simulink model "PrinterILC_exp"  (Simulink 7.8)
settings: Solver=FixedStepDiscrete  StartTime=0.0  StopTime=30  FixedStep=1/1000  RelTol=1e-3
undefined symbols (not defined in the file or in its folder): DiscIntNeverNeededParam
libraries: simulink x3
settings Model: Creator=root  LastModifiedBy=root  SimulationMode=external  ExtModeAutoUpdateStatusClock=off
settings DataIOCC: SaveOutput=off  SignalLogging=off  DSMLogging=off  SaveTime=off
settings OptimizationCC: InitFltsAndDblsToZero=on
settings DebuggingCC: SaveWithParameterizedLinksMsg=none  SignalResolutionControl=TryResolveAllWithWarning  MultiTaskDSMMsg=warning  MultiTaskCondExecSysMsg=none  FcnCallInpInsideContextMsg=Use local settings  StrictBusMsg=None
settings SFSimCC: SFSimEcho=off  SimBuildMode=sf_nonincremental_build
settings RTWCC: SystemTargetFile=ectarget.tlc  MakeCommand="make_rtw OPTS=\"-DNETIF_ID=0\""  TemplateMakefile=ec_unix.tmf  Description=Ethercattarget Real-Time Target for PREEMPT-RT/Linux  ProcessScript=ectarget_make_rtw_hook  IncludeERTFirstTime=on  RTWCompilerOptimization=On
settings CodeAppCC: GenerateComments=off  SimulinkBlockComments=off
settings GRTTargetCC: TargetFcnLib=ansi_tfl_tmw.mat  ExtMode=on

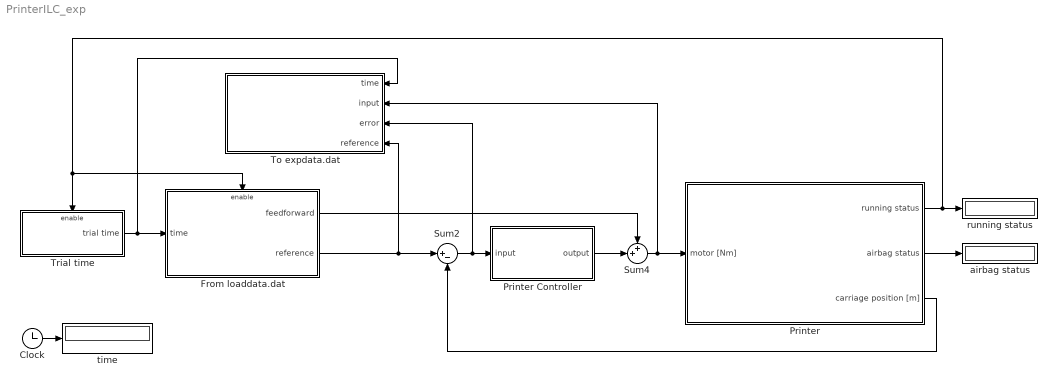
== system PrinterILC_exp ==
  Clock : Clock
  From loaddata.dat : Subsystem
  Printer : Subsystem
  Printer Controller : Subsystem
  Sum2 : Sum  Inputs=|+-
  Sum4 : Sum  Inputs=++|  SaturateOnIntegerOverflow=on  InputSameDT=on  OutDataTypeStr=Inherit: Same as first input
  To expdata.dat : Subsystem
  Trial time : Subsystem  TreatAsAtomicUnit=on
  airbag status : Display
      settings: Decimation=50
  running status : Display
      settings: Decimation=50
  time : Display
      settings: Decimation=50
  wires:
  Sum2/1 -> To expdata.dat/3(error), Printer Controller/1(input)
  From loaddata.dat/2(reference) -> Sum2/1, To expdata.dat/4(reference)
  Clock/1 -> time/1
  Printer/3(carriage position [m]) -> Sum2/2
  Printer Controller/1(output) -> Sum4/2
  From loaddata.dat/1(feedforward) -> Sum4/1
  Sum4/1 -> Printer/1(motor [Nm]), To expdata.dat/2(input)
  Printer/1(running status) -> Trial time/Enable, From loaddata.dat/Enable, running status/1
  Trial time/1(trial time) -> From loaddata.dat/1(time), To expdata.dat/1(time)
  Printer/2(airbag status) -> airbag status/1

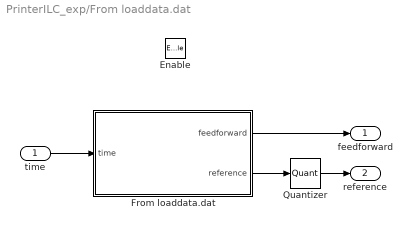
== system PrinterILC_exp/From loaddata.dat ==
  time : Inport
  Enable : EnablePort  StatesWhenEnabling=reset
  From loaddata.dat : Subsystem
  Quantizer : Quantizer  QuantizationInterval=1/(600*100/2.54)
  feedforward : Outport
  reference : Outport  Port=2
  wires:
  time/1 -> From loaddata.dat/1(time)
  From loaddata.dat/1(feedforward) -> feedforward/1
  From loaddata.dat/2(reference) -> Quantizer/1
  Quantizer/1 -> reference/1

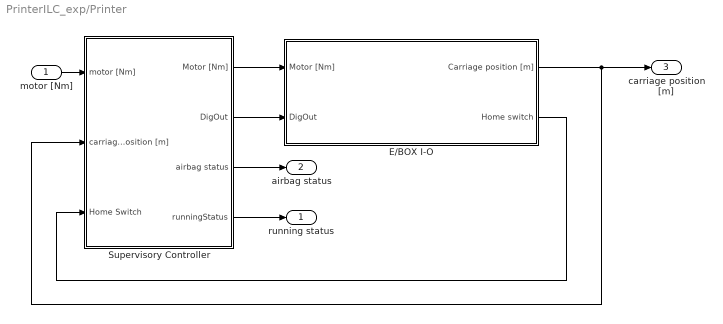
== system PrinterILC_exp/Printer ==
  motor [Nm] : Inport
  E/BOX I-O : Subsystem
  Supervisory Controller : Subsystem
  running status : Outport
  airbag status : Outport  Port=2
  carriage position [m] : Outport  Port=3
  wires:
  E/BOX I-O/1(Carriage position [m]) -> Supervisory Controller/2(carriage position [m]), carriage position [m]/1
  Supervisory Controller/1(Motor [Nm]) -> E/BOX I-O/1(Motor [Nm])
  E/BOX I-O/2(Home switch) -> Supervisory Controller/3(Home Switch)
  motor [Nm]/1 -> Supervisory Controller/1(motor [Nm])
  Supervisory Controller/3(airbag status) -> airbag status/1
  Supervisory Controller/4(runningStatus) -> running status/1
  Supervisory Controller/2(DigOut) -> E/BOX I-O/2(DigOut)

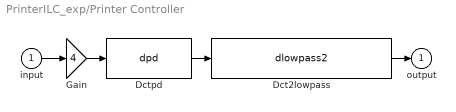
== system PrinterILC_exp/Printer Controller ==
  input : Inport
  Dct2lowpass : S-Function  FunctionName=dlowpass2  Parameters=f_den, b_den, 0.001  EnableBusSupport=off  mask(dctools){f_den=40, b_den=0.7}
      mask prompts: f_den "Pole [Hz]"; b_den "Damping pole [-]"
      mask help: This block implements a discrete time 2nd order lowpass filter.
      mask Display: disp('DCT 2nd order lowpass')
  Dctpd : S-Function  FunctionName=dpd  Parameters=kp, kv, 0.001  EnableBusSupport=off  mask(dctools){kp=40, kv=1}
      mask help: This block implements a discrete time pd filter.
      mask Display: disp('DCT pd')
  Gain : Gain  Gain=4  SaturateOnIntegerOverflow=on  OutDataTypeStr=Inherit: Same as input  ParamDataTypeStr=Inherit: Same as input
  output : Outport
  wires:
  input/1 -> Gain/1
  Gain/1 -> Dctpd/1
  Dctpd/1 -> Dct2lowpass/1
  Dct2lowpass/1 -> output/1

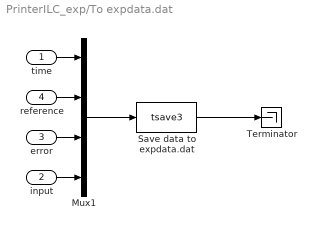
== system PrinterILC_exp/To expdata.dat ==
  time : Inport
  input : Inport  Port=2
  error : Inport  Port=3
  reference : Inport  Port=4
  Mux1 : Mux
  Save data to expdata.dat : S-Function  FunctionName=tsave3  Parameters=0  EnableBusSupport=off
  Terminator : Terminator
  wires:
  Mux1/1 -> Save data to expdata.dat/1
  Save data to expdata.dat/1 -> Terminator/1
  time/1 -> Mux1/1
  input/1 -> Mux1/4
  error/1 -> Mux1/3
  reference/1 -> Mux1/2

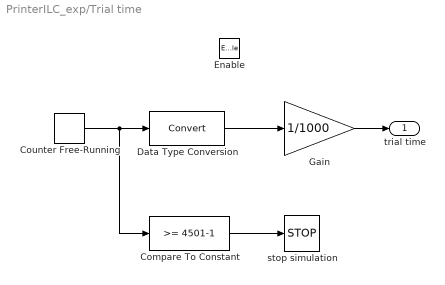
== system PrinterILC_exp/Trial time ==
  Enable : EnablePort  StatesWhenEnabling=reset
  Compare To Constant : simulink/Logic and Bit Operations/Compare To Constant  relop=>=  const=4501-1  OutDataTypeStr=boolean
  Counter Free-Running : simulink/Sources/Counter Free-Running  NumBits=32  tsamp=-1
  Data Type Conversion : DataTypeConversion
  Gain : Gain  Gain=1/1000
  stop simulation : Stop
  trial time : Outport  InitialOutput=0
  wires:
  Counter Free-Running/1 -> Compare To Constant/1, Data Type Conversion/1
  Compare To Constant/1 -> stop simulation/1
  Data Type Conversion/1 -> Gain/1
  Gain/1 -> trial time/1

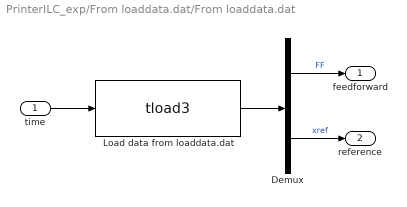
== system PrinterILC_exp/From loaddata.dat/From loaddata.dat ==
  time : Inport
  Demux : Demux  Outputs=2
  Load data from loaddata.dat : S-Function  FunctionName=tload3  Parameters=0  EnableBusSupport=off
  feedforward : Outport
  reference : Outport  Port=2
  wires:
  time/1 -> Load data from loaddata.dat/1
  Load data from loaddata.dat/1 -> Demux/1
  Demux/1 -> feedforward/1  "FF"
  Demux/2 -> reference/1  "xref"

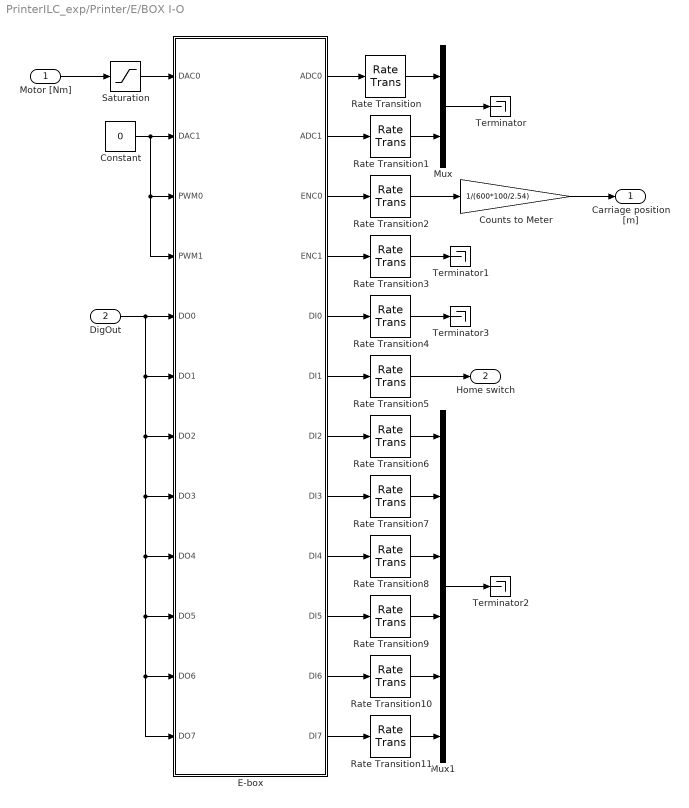
== system PrinterILC_exp/Printer/E/BOX I-O ==
  Motor [Nm] : Inport
  DigOut : Inport  Port=2
  Constant : Constant  Value=0
  Counts to Meter : Gain  Gain=1/(600*100/2.54)
  E-box : Subsystem  mask(E-box){link_id=0}
      mask prompts: link_id "Link id (>=0)"
  Mux : Mux  Inputs=2
  Mux1 : Mux  Inputs=6
  Rate Transition{,1..11} (12 alike) : RateTransition
  Saturation : Saturate  UpperLimit=2.5  LowerLimit=-2.5
  Terminator{,1..3} (4 alike) : Terminator
  Carriage position [m] : Outport
  Home switch : Outport  Port=2
  wires:
  E-box/3(ENC0) -> Rate Transition2/1
  Counts to Meter/1 -> Carriage position [m]/1
  DigOut/1 -> E-box/12(DO7), E-box/11(DO6), E-box/10(DO5), E-box/9(DO4), E-box/8(DO3), E-box/7(DO2), E-box/6(DO1), E-box/5(DO0)
  E-box/1(ADC0) -> Rate Transition/1
  E-box/2(ADC1) -> Rate Transition1/1
  Mux/1 -> Terminator/1
  Motor [Nm]/1 -> Saturation/1
  E-box/4(ENC1) -> Rate Transition3/1
  E-box/5(DI0) -> Rate Transition4/1
  E-box/6(DI1) -> Rate Transition5/1
  E-box/7(DI2) -> Rate Transition6/1
  E-box/8(DI3) -> Rate Transition7/1
  E-box/9(DI4) -> Rate Transition8/1
  E-box/10(DI5) -> Rate Transition9/1
  E-box/11(DI6) -> Rate Transition10/1
  E-box/12(DI7) -> Rate Transition11/1
  Rate Transition/1 -> Mux/1
  Rate Transition1/1 -> Mux/2
  Rate Transition2/1 -> Counts to Meter/1
  Rate Transition3/1 -> Terminator1/1
  Rate Transition4/1 -> Terminator3/1
  Rate Transition5/1 -> Home switch/1
  Rate Transition6/1 -> Mux1/1
  Rate Transition7/1 -> Mux1/2
  Rate Transition8/1 -> Mux1/3
  Rate Transition9/1 -> Mux1/4
  Rate Transition10/1 -> Mux1/5
  Rate Transition11/1 -> Mux1/6
  Saturation/1 -> E-box/1(DAC0)
  Mux1/1 -> Terminator2/1
  Constant/1 -> E-box/3(PWM0), E-box/4(PWM1), E-box/2(DAC1)

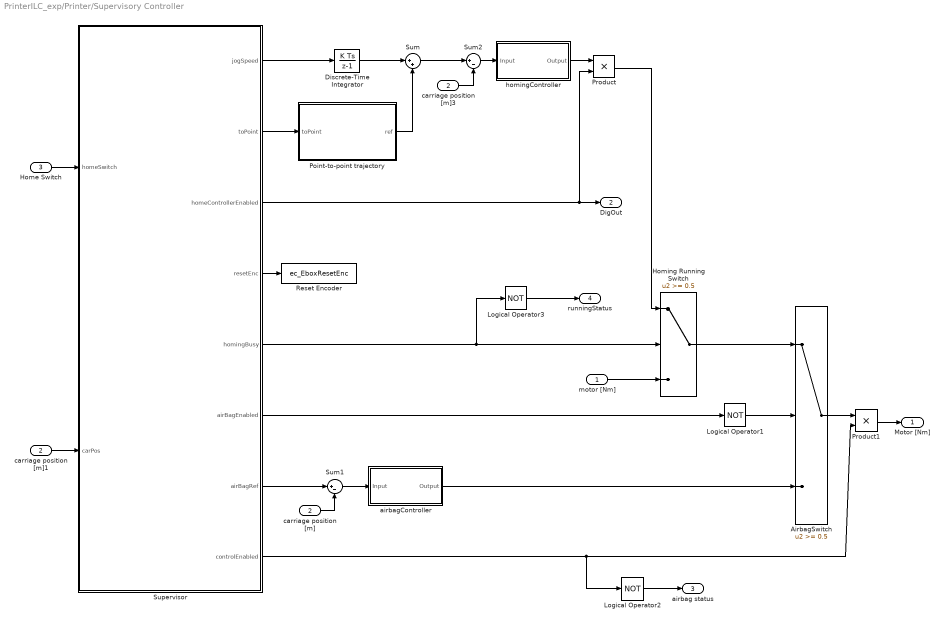
== system PrinterILC_exp/Printer/Supervisory Controller ==
  motor [Nm] : Inport
  carriage position [m] : Inport  Port=2
  Home Switch : Inport  Port=3
  AirbagSwitch : Switch  Threshold=0.5
  Discrete-Time Integrator : DiscreteIntegrator  SampleTime=-1  ICPrevOutput=DiscIntNeverNeededParam  ICPrevScaledInput=DiscIntNeverNeededParam
  Homing Running Switch : Switch  Threshold=0.5
  Logical Operator1 : Logic  Operator=NOT  AllPortsSameDT=off  OutDataTypeStr=boolean
  Logical Operator2 : Logic  Operator=NOT  AllPortsSameDT=off  OutDataTypeStr=boolean
  Logical Operator3 : Logic  Operator=NOT  AllPortsSameDT=off  OutDataTypeStr=boolean
  Point-to-point trajectory : Subsystem
  Product : Product  RndMeth=Zero
  Product1 : Product  RndMeth=Zero
  Reset Encoder : S-Function  FunctionName=ec_EboxResetEnc  Parameters=link_id  EnableBusSupport=off  mask{link_id=0}
      mask prompts: link_id "analog in id (start from 1)"
  Sum : Sum  Inputs=|++
  Sum1 : Sum  Inputs=|+-
  Sum2 : Sum  Inputs=|+-
  Supervisor : Stateflow chart  TreatAsAtomicUnit=on
  airbagController : Subsystem
  carriage position [m]1 : InportShadow  Port=2
  carriage position [m]3 : InportShadow  Port=2
  homingController : Subsystem
  Motor [Nm] : Outport
  DigOut : Outport  Port=2
  airbag status : Outport  Port=3
  runningStatus : Outport  Port=4
  wires:
  Homing Running Switch/1 -> AirbagSwitch/1
  Sum/1 -> Sum2/1
  Sum2/1 -> homingController/1(Input)
  Home Switch/1 -> Supervisor/1(homeSwitch)
  Supervisor/1(jogSpeed) -> Discrete-Time Integrator/1
  carriage position [m]3/1 -> Sum2/2
  motor [Nm]/1 -> Homing Running Switch/3
  homingController/1(Output) -> Product/1
  Product/1 -> Homing Running Switch/1
  Discrete-Time Integrator/1 -> Sum/1
  Point-to-point trajectory/1(ref) -> Sum/2
  Supervisor/5(homingBusy) -> Homing Running Switch/2, Logical Operator3/1
  Supervisor/3(homeControllerEnabled) -> DigOut/1, Product/2
  Supervisor/2(toPoint) -> Point-to-point trajectory/1(toPoint)
  Supervisor/4(resetEnc) -> Reset Encoder/1
  carriage position [m]1/1 -> Supervisor/2(carPos)
  Supervisor/6(airBagEnabled) -> Logical Operator1/1
  Logical Operator1/1 -> AirbagSwitch/2
  airbagController/1(Output) -> AirbagSwitch/3
  Sum1/1 -> airbagController/1(Input)
  carriage position [m]/1 -> Sum1/2
  Supervisor/7(airBagRef) -> Sum1/1
  AirbagSwitch/1 -> Product1/1
  Product1/1 -> Motor [Nm]/1
  Supervisor/8(controlEnabled) -> Product1/2, Logical Operator2/1
  Logical Operator2/1 -> airbag status/1
  Logical Operator3/1 -> runningStatus/1

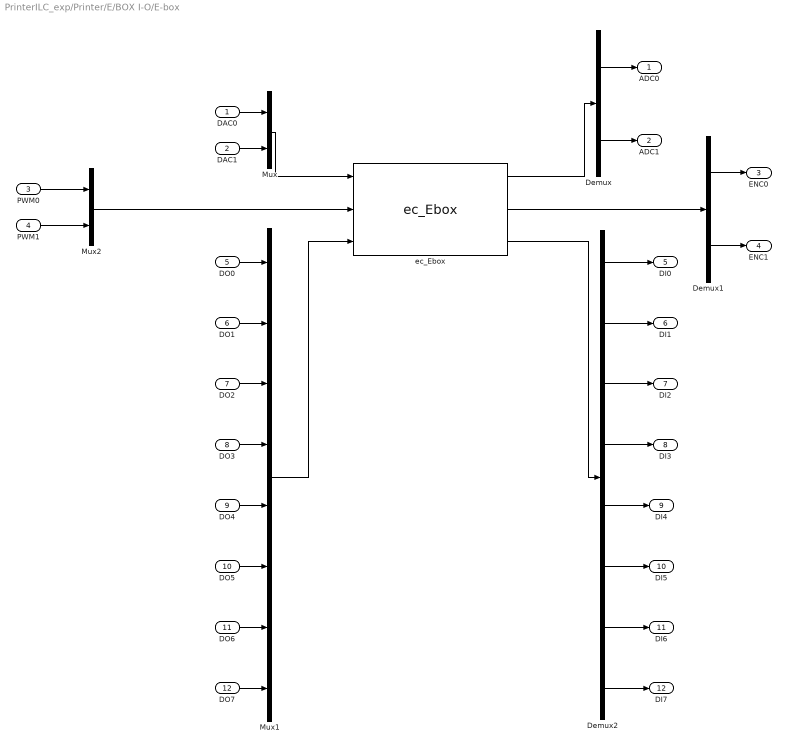
== system PrinterILC_exp/Printer/E/BOX I-O/E-box ==
  DAC0 : Inport
  DAC1 : Inport  Port=2
  PWM0 : Inport  Port=3
  PWM1 : Inport  Port=4
  DO0 : Inport  Port=5
  DO1 : Inport  Port=6
  DO2 : Inport  Port=7
  DO3 : Inport  Port=8
  DO4 : Inport  Port=9
  DO5 : Inport  Port=10
  DO6 : Inport  Port=11
  DO7 : Inport  Port=12
  Demux : Demux  Outputs=2
  Demux1 : Demux  Outputs=2
  Demux2 : Demux  Outputs=8
  Mux : Mux  Inputs=2
  Mux1 : Mux  Inputs=8
  Mux2 : Mux  Inputs=2
  ec_Ebox : S-Function  FunctionName=ec_Ebox  Parameters=link_id  EnableBusSupport=off  mask{link_id=link_id}
      mask prompts: link_id "analog in id (start from 1)"
      mask Display:
      | port_label('output',1,'ADC')
      | port_label('output',2,'ENC')
      | port_label('output',3,'DI')
      | port_label('input',1,'DAC')
      | port_label('input',2,'PWM')
      | port_label('input',3,'DO')
  ADC0 : Outport
  ADC1 : Outport  Port=2
  ENC0 : Outport  Port=3
  ENC1 : Outport  Port=4
  DI0 : Outport  Port=5
  DI1 : Outport  Port=6
  DI2 : Outport  Port=7
  DI3 : Outport  Port=8
  DI4 : Outport  Port=9
  DI5 : Outport  Port=10
  DI6 : Outport  Port=11
  DI7 : Outport  Port=12
  wires:
  ec_Ebox/1 -> Demux/1
  Demux/1 -> ADC0/1
  Demux/2 -> ADC1/1
  Demux1/1 -> ENC0/1
  Demux1/2 -> ENC1/1
  ec_Ebox/2 -> Demux1/1
  Mux/1 -> ec_Ebox/1
  DAC0/1 -> Mux/1
  DAC1/1 -> Mux/2
  ec_Ebox/3 -> Demux2/1
  Demux2/1 -> DI0/1
  Demux2/2 -> DI1/1
  Demux2/3 -> DI2/1
  Demux2/4 -> DI3/1
  Demux2/5 -> DI4/1
  Demux2/6 -> DI5/1
  Demux2/7 -> DI6/1
  Demux2/8 -> DI7/1
  DO0/1 -> Mux1/1
  DO1/1 -> Mux1/2
  DO2/1 -> Mux1/3
  DO3/1 -> Mux1/4
  DO4/1 -> Mux1/5
  DO5/1 -> Mux1/6
  DO6/1 -> Mux1/7
  DO7/1 -> Mux1/8
  Mux1/1 -> ec_Ebox/3
  Mux2/1 -> ec_Ebox/2
  PWM0/1 -> Mux2/1
  PWM1/1 -> Mux2/2

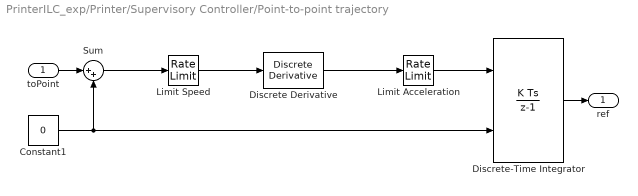
== system PrinterILC_exp/Printer/Supervisory Controller/Point-to-point trajectory ==
  toPoint : Inport
  Constant1 : Constant  Value=0
  Discrete Derivative : simulink/Discrete/Discrete Derivative  gainval=1.0  ICPrevScaledInput=0.0  InputProcessing=Inherited  OutMin=[]  OutMax=[]  OutDataType=fixdt(1, 16)  OutScaling=2^-10  DoSatur=off
  Discrete-Time Integrator : DiscreteIntegrator  InitialConditionSource=external  SampleTime=-1  ICPrevOutput=DiscIntNeverNeededParam  ICPrevScaledInput=DiscIntNeverNeededParam
  Limit Acceleration : RateLimiter  RisingSlewLimit=0.5  FallingSlewLimit=-0.5  SampleTimeMode=inherited
  Limit Speed : RateLimiter  RisingSlewLimit=0.1  FallingSlewLimit=-0.1  SampleTimeMode=inherited
  Sum : Sum  Inputs=|++
  ref : Outport
  wires:
  Sum/1 -> Limit Speed/1
  Constant1/1 -> Sum/2, Discrete-Time Integrator/2
  Limit Acceleration/1 -> Discrete-Time Integrator/1
  Discrete Derivative/1 -> Limit Acceleration/1
  Limit Speed/1 -> Discrete Derivative/1
  toPoint/1 -> Sum/1
  Discrete-Time Integrator/1 -> ref/1

== system PrinterILC_exp/Printer/Supervisory Controller/airbagController ==
  Input : Inport
  Dct2lowpass3 : S-Function  FunctionName=dlowpass2  Parameters=f_den, b_den, 0.001  EnableBusSupport=off  mask(dctools){f_den=40, b_den=0.7}
      mask prompts: f_den "Pole [Hz]"; b_den "Damping pole [-]"
      mask help: This block implements a discrete time 2nd order lowpass filter.
      mask Display: disp('DCT 2nd order lowpass')
  Dctpd2 : S-Function  FunctionName=dpd  Parameters=kp, kv, 0.001  EnableBusSupport=off  mask(dctools){kp=40, kv=1}
      mask help: This block implements a discrete time pd filter.
      mask Display: disp('DCT pd')
  Gain1 : Gain  Gain=4  SaturateOnIntegerOverflow=on  OutDataTypeStr=Inherit: Same as input  ParamDataTypeStr=Inherit: Same as input
  Output : Outport
  wires:
  Input/1 -> Gain1/1
  Gain1/1 -> Dctpd2/1
  Dctpd2/1 -> Dct2lowpass3/1
  Dct2lowpass3/1 -> Output/1

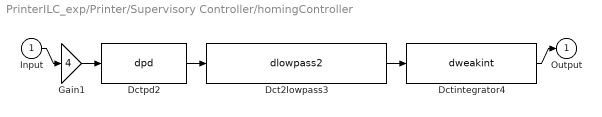
== system PrinterILC_exp/Printer/Supervisory Controller/homingController ==
  Input : Inport
  Dct2lowpass3 : S-Function  FunctionName=dlowpass2  Parameters=f_den, b_den, 0.001  EnableBusSupport=off  mask(dctools){f_den=40, b_den=0.7}
      mask prompts: f_den "Pole [Hz]"; b_den "Damping pole [-]"
      mask help: This block implements a discrete time 2nd order lowpass filter.
      mask Display: disp('DCT 2nd order lowpass')
  Dctintegrator4 : S-Function  FunctionName=dweakint  Parameters=f_num, 0.001  EnableBusSupport=off  mask(dctools){f_num=0.25}
      mask prompts: f_num "Zero [Hz]"
      mask help: This block implements a discrete time weak integrator filter.
      mask Display: disp('DCT integrator')
  Dctpd2 : S-Function  FunctionName=dpd  Parameters=kp, kv, 0.001  EnableBusSupport=off  mask(dctools){kp=40, kv=1}
      mask help: This block implements a discrete time pd filter.
      mask Display: disp('DCT pd')
  Gain1 : Gain  Gain=4  SaturateOnIntegerOverflow=on  OutDataTypeStr=Inherit: Same as input  ParamDataTypeStr=Inherit: Same as input
  Output : Outport
  wires:
  Input/1 -> Gain1/1
  Gain1/1 -> Dctpd2/1
  Dctpd2/1 -> Dct2lowpass3/1
  Dct2lowpass3/1 -> Dctintegrator4/1
  Dctintegrator4/1 -> Output/1

== stateflow chart Printer/Supervisory Controller/Supervisor ==
  state AirbagLeft
    entry:
    airBagEnabled = 1;
    airBagRef=-0.01;
  state DisableOutputs
    entry:
    controlEnabled=0;
  state Homing
    entry:
    %Set jog speed and homing state
    toPoint = 0;
    homingBusy = 1;
    jogSpeed = -0.1;
    homeControllerEnabled=1;
  state AirbagRight
    entry:
    airBagEnabled = 1;
    airBagRef=0.35;
  state EnableRunAndSafety
    entry:
    resetEnc=0;
    homingBusy=0;
  state MovetoX0
    entry:
    jogSpeed = 0.0;
    toPoint = 0.04;
  state ResetEnc
    entry:
    resetEnc=1;
  state DisableControl
    entry:
    homeControllerEnabled=0;
  (default) -> Homing
  AirbagLeft -> DisableOutputs : after(1,sec)
  AirbagRight -> DisableOutputs : after(1,sec)
  EnableRunAndSafety -> AirbagLeft [order 1] : [carPos<-0.01]
  Homing -> MovetoX0 : %Transition if homeswitch becomes high
      | [homeSwitch]
  EnableRunAndSafety -> AirbagRight [order 2] : [carPos>0.35]
  ResetEnc -> EnableRunAndSafety : after(0.1,sec)
  MovetoX0 -> DisableControl : %Allow time for moving
      | after(0.5,sec)
  DisableControl -> ResetEnc : %Allow settling of belt
      | after(0.5,sec)
  data: jogSpeed output double; toPoint output double; homeControllerEnabled output double; resetEnc output double; homingBusy output double =1; homeSwitch input double; carPos input double; airBagEnabled output double =0; airBagRef output double =0; controlEnabled output double =1
